simulink model "sistema_lti_simplificado"  (R2019a)
settings: Solver=ode45  StartTime=0.0  StopTime=10.0  MaxStep=1e-6  RelTol=1e-6
values from neighbouring files (symbols this model uses):
  b_eq = b_m + b_l/r^2    (= 1.5e-05)    [parametros_de_sistema.m]    (also in sistema_completo_nl_script.m)
  dT_l = 6.28    [parametros_de_sistema.m]    (also in sistema_completo_nl_script.m)
  J_eq = J_m + J_l/r^2    (= 5.65099476805e-06)    [parametros_de_sistema.m]    (also in sistema_completo_nl_script.m)
  L_q = 5.8e-3    (= 0.0058)    [parametros_de_sistema.m]    (also in sistema_completo_nl_script.m)
  lambda_m = 0.01546    [parametros_de_sistema.m]    (also in sistema_completo_nl_script.m)
  P_p = 3    [parametros_de_sistema.m]    (also in sistema_completo_nl_script.m)
  r = 314.3008    [parametros_de_sistema.m]    (also in sistema_completo_nl_script.m)
  R_s_prom = (1.32 - 1.02)/2    (= 0.15)    [parametros_de_sistema.m]
libraries: eeTransforms x1
settings Model: Creator=pedro  LastModifiedBy=pedro

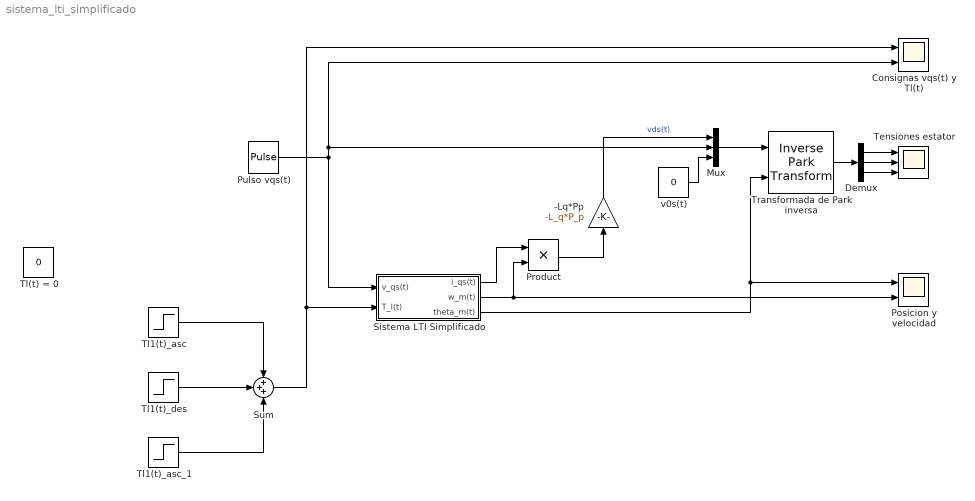
== system sistema_lti_simplificado ==
  -Lq*Pp : Gain  Gain=-L_q*P_p
  Consignas vqs(t) y Tl(t) : Scope  NumInputPorts=2
  Demux : Demux  Outputs=3
  Mux : Mux  Inputs=3
  Posicion y velocidad : Scope  NumInputPorts=2
  Product : Product
  Pulso vqs(t) : DiscretePulseGenerator  PulseType=Time based  Amplitude=19.596  Period=3  PulseWidth=20  PhaseDelay=0.1
  Sistema LTI Simplificado : Subsystem
  Sum : Sum  Inputs=+++
  Tensiones estator : Scope  NumInputPorts=3
  Tl(t) = 0 : Constant  Value=0
  Tl1(t)_asc : Step  Time=0  After=dT_l  SampleTime=0
  Tl1(t)_asc_1 : Step  Time=0.9  After=dT_l  SampleTime=0
  "Tl1(t)_des " : Step  Time=0.3  After=-2*dT_l  SampleTime=0
  "Transformada de Park inversa " : eeTransforms/Inverse Park Transform  AxisAlignment=Q-axis  PowerInvariant=off
      settings: SourceProductName=Simscape Electrical
  v0s(t) : Constant  Value=0
  wires:
  Tl1(t)_asc_1/1 -> Sum/3
  Sum/1 -> Consignas vqs(t) y Tl(t)/1, Sistema LTI Simplificado/2("T_l(t) ")
  Tl1(t)_asc/1 -> Sum/1
  "Tl1(t)_des "/1 -> Sum/2
  Demux/3 -> Tensiones estator/3
  Sistema LTI Simplificado/2(w_m(t)) -> Product/2, Posicion y velocidad/2
  v0s(t)/1 -> Mux/3
  "Transformada de Park inversa "/1 -> Demux/1
  Sistema LTI Simplificado/3(theta_m(t)) -> Posicion y velocidad/1, "Transformada de Park inversa "/2
  Mux/1 -> "Transformada de Park inversa "/1
  Pulso vqs(t)/1 -> Consignas vqs(t) y Tl(t)/2, Mux/2, Sistema LTI Simplificado/1(v_qs(t))
  Demux/1 -> Tensiones estator/1
  Demux/2 -> Tensiones estator/2
  Sistema LTI Simplificado/1("i_qs(t) ") -> Product/1
  Product/1 -> -Lq*Pp/1
  -Lq*Pp/1 -> Mux/1  "vds(t)"

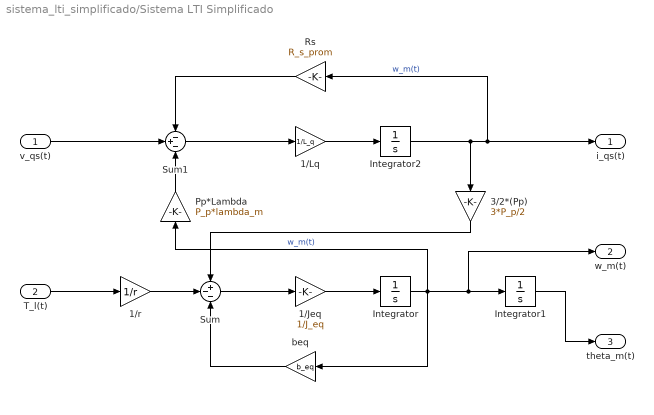
== system sistema_lti_simplificado/Sistema LTI Simplificado ==
  v_qs(t) : Inport
  "T_l(t) " : Inport  Port=2
  "1/Jeq " : Gain  Gain=1/J_eq
  1/Lq : Gain  Gain=1/L_q
  1/r : Gain  Gain=1/r
  3/2*(Pp) : Gain  Gain=3*P_p/2
  Integrator : Integrator
  Integrator1 : Integrator
  Integrator2 : Integrator
  Pp*Lambda : Gain  Gain=P_p*lambda_m
  Rs : Gain  Gain=R_s_prom
  Sum : Sum  Inputs=+--
  Sum1 : Sum  Inputs=-+-
  beq : Gain  Gain=b_eq
  "i_qs(t) " : Outport
  w_m(t) : Outport  Port=2
  theta_m(t) : Outport  Port=3
  wires:
  1/r/1 -> Sum/2
  "T_l(t) "/1 -> 1/r/1
  Sum/1 -> "1/Jeq "/1
  "1/Jeq "/1 -> Integrator/1
  Integrator/1 -> Pp*Lambda/1, beq/1, w_m(t)/1, Integrator1/1  "w_m(t)"
  beq/1 -> Sum/3
  v_qs(t)/1 -> Sum1/2
  Sum1/1 -> 1/Lq/1
  Pp*Lambda/1 -> Sum1/3
  1/Lq/1 -> Integrator2/1
  Integrator2/1 -> Rs/1, "i_qs(t) "/1, 3/2*(Pp)/1  "w_m(t)"
  Rs/1 -> Sum1/1
  3/2*(Pp)/1 -> Sum/1
  Integrator1/1 -> theta_m(t)/1
